simulink model "rc_coder"  (R2019b)
settings: Solver=FixedStepDiscrete  StartTime=0.0  StopTime=Inf  FixedStep=0.025  RelTol=1e-3  EnableMultiTasking=on
PreLoadFcn:
  | mdlname = bdroot;
  | oldFolder = cd(fileparts(which(mdlname)));
  | % cd ..\
  | 
  | load('./bus_type/bus_type.mat');
model workspace (MAT data in the model file):
  ADCDRES = Simulink.Parameter
  ADCDRES.Value = 65536
  ADCDRES.DataType = 'auto'
  ADCDRES.Dimensions = [1 1]
  ADCSRES = Simulink.Parameter
  ADCSRES.Value = 4096
  ADCSRES.DataType = 'auto'
  ADCSRES.Dimensions = [1 1]
  CLK = Simulink.Parameter
  CLK.Value = 200000000
  CLK.DataType = 'auto'
  CLK.Dimensions = [1 1]
  EncoderScaler = Simulink.Parameter
  EncoderScaler.Value = 1000
  EncoderScaler.DataType = 'auto'
  EncoderScaler.Dimensions = [1 1]
  GearBoxScaler = Simulink.Parameter
  GearBoxScaler.Value = 1
  GearBoxScaler.DataType = 'auto'
  GearBoxScaler.Dimensions = [1 1]
  Kd_T = Simulink.Parameter
  Kd_T.Value = 0.02
  Kd_T.DataType = 'auto'
  Kd_T.Dimensions = [1 1]
  Kd_theta = Simulink.Parameter
  Kd_theta.Value = 0
  Kd_theta.DataType = 'auto'
  Kd_theta.Dimensions = [1 1]
  Ki_T = Simulink.Parameter
  Ki_T.Value = 0
  Ki_T.DataType = 'auto'
  Ki_T.Dimensions = [1 1]
  Ki_theta = Simulink.Parameter
  Ki_theta.Value = 0.1
  Ki_theta.DataType = 'auto'
  Ki_theta.Dimensions = [1 1]
  Kp_T = Simulink.Parameter
  Kp_T.Value = 0.1
  Kp_T.DataType = 'auto'
  Kp_T.Dimensions = [1 1]
  Kp_theta = Simulink.Parameter
  Kp_theta.Value = 4
  Kp_theta.DataType = 'auto'
  Kp_theta.Dimensions = [1 1]
  LowerTempLimitHigh = Simulink.Parameter
  LowerTempLimitHigh.Value = 30
  LowerTempLimitHigh.DataType = 'auto'
  LowerTempLimitHigh.Dimensions = [1 1]
  LowerTempLimitLow = Simulink.Parameter
  LowerTempLimitLow.Value = 15
  LowerTempLimitLow.DataType = 'auto'
  LowerTempLimitLow.Dimensions = [1 1]
  MinMeasurableSpd = Simulink.Parameter
  MinMeasurableSpd.Value = 2
  MinMeasurableSpd.DataType = 'auto'
  MinMeasurableSpd.Dimensions = [1 1]
  ModePWM = Simulink.Parameter
  ModePWM.Value = 56
  ModePWM.DataType = 'single'
  ModePWM.Dimensions = [1 1]
  ModePosition = Simulink.Parameter
  ModePosition.Value = 53
  ModePosition.DataType = 'single'
  ModePosition.Dimensions = [1 1]
  ModePrecool = Simulink.Parameter
  ModePrecool.Value = 60
  ModePrecool.DataType = 'single'
  ModePrecool.Dimensions = [1 1]
  ModeTemp = Simulink.Parameter
  ModeTemp.Value = 55
  ModeTemp.DataType = 'single'
  ModeTemp.Dimensions = [1 1]
  PWMFreq = Simulink.Parameter
  PWMFreq.Value = 20
  PWMFreq.DataType = 'auto'
  PWMFreq.Dimensions = [1 1]
  QuadratureEncScaler = Simulink.Parameter
  QuadratureEncScaler.Value = 4
  QuadratureEncScaler.DataType = 'auto'
  QuadratureEncScaler.Dimensions = [1 1]
  S1DelaySeconds = Simulink.Parameter
  S1DelaySeconds.Value = 1
  S1DelaySeconds.DataType = 'auto'
  S1DelaySeconds.Dimensions = [1 1]
  S2DelaySeconds = Simulink.Parameter
  S2DelaySeconds.Value = 2
  S2DelaySeconds.DataType = 'auto'
  S2DelaySeconds.Dimensions = [1 1]
  S3DelaySeconds = Simulink.Parameter
  S3DelaySeconds.Value = 3
  S3DelaySeconds.DataType = 'auto'
  S3DelaySeconds.Dimensions = [1 1]
  S4DelaySeconds = Simulink.Parameter
  S4DelaySeconds.Value = 4
  S4DelaySeconds.DataType = 'auto'
  S4DelaySeconds.Dimensions = [1 1]
  SamplingR = Simulink.Parameter
  SamplingR.Value = 0.1
  SamplingR.DataType = 'auto'
  SamplingR.Dimensions = [1 1]
  StepSize = Simulink.Parameter
  StepSize.Value = 0.025
  StepSize.DataType = 'auto'
  StepSize.Dimensions = [1 1]
  TErrBand = Simulink.Parameter
  TErrBand.Value = 0.2
  TErrBand.DataType = 'auto'
  TErrBand.Dimensions = [1 1]
  ThetaErrBand = Simulink.Parameter
  ThetaErrBand.Value = 0.2
  ThetaErrBand.DataType = 'auto'
  ThetaErrBand.Dimensions = [1 1]
  VADCREF = Simulink.Parameter
  VADCREF.Value = 3
  VADCREF.DataType = 'auto'
  VADCREF.Dimensions = [1 1]
undefined symbols (not defined in the file or in its folder): DiscIntNeverNeededParam, Down, GPTRIP1SEL, GPTRIP2SEL, TZ1, TZ2, Up
libraries: simulink x21, c2802xlib x12, c2837xDlib x10, c280xlib x9, dspstat3 x8, dspfdesign x7, commutil2 x3, c2000lib x2
(part 1 of 4)
CloseFcn:
  | cd(oldFolder);
Description:
  | -> System Description <-
  | - Development environment:
  |     Matlab (version 2019b) with licence to
  |     - Simulink
  |     - Embedded Coder Support Package for Texas Instruments C2000 Processors
  |     - StateFlow
  | - Control board:
  |     TI LAUNCHXL F28379D
settings Model: SimulationMode=external  ExtModeTrigDuration=8  OrderedModelArguments=off  Creator=Quinn Ding  LastModifiedBy=Quinn
settings OptimizationCC: DefaultUnderspecifiedDataType=single  EnhancedBackFolding=on  PassReuseOutputArgsAs=Individual arguments  ZeroExternalMemoryAtStartup=off  MaxStackSize=1024  OptimizeBlockOrder=speed  DifferentSizesBufferReuse=on  OptimizationCustomize=off  DenormalBehavior=FlushToZero  EfficientTunableParamExpr=on
settings DebuggingCC: ParameterTunabilityLossMsg=error
settings HardwareCC: ProdBitPerChar=16  ProdBitPerInt=16  ProdBitPerPointer=32  ProdBitPerSizeT=32  ProdBitPerPtrDiffT=32  ProdLargestAtomicInteger=Integer  ProdLargestAtomicFloat=None  ProdWordSize=16  ProdLongLongMode=on  ProdHWDeviceType=Texas Instruments->C2000
settings SFSimCC: MATLABDynamicMemAlloc=off
settings RTWCC: SystemTargetFile=ert.tlc  HardwareBoard=TI Delfino F28379D LaunchPad  TLCOptions=-aInlineSetEventsForThisBaseRateFcn=TLC_FALSE -aSuppressMultiTaskScheduler=TLC_FALSE -aRateBasedStepFcn=1  TemplateMakefile=ert_default_tmf  Toolchain=Texas Instruments Code Composer Studio (C2000)  BuildConfiguration=Faster Runs  IncludeHyperlinkInReport=on
settings CodeAppCC: ForceParamTrailComments=on  IgnoreCustomStorageClasses=off  OperatorAnnotations=on  SimulinkDataObjDesc=on  SFDataObjDesc=on  InsertBlockDesc=on
settings ERTTargetCC: TargetLangStandard=C99 (ISO)  CodeReplacementLibrary=TI C28x  ExtModeStaticAllocSize=10000  RootIOFormat=Structure reference

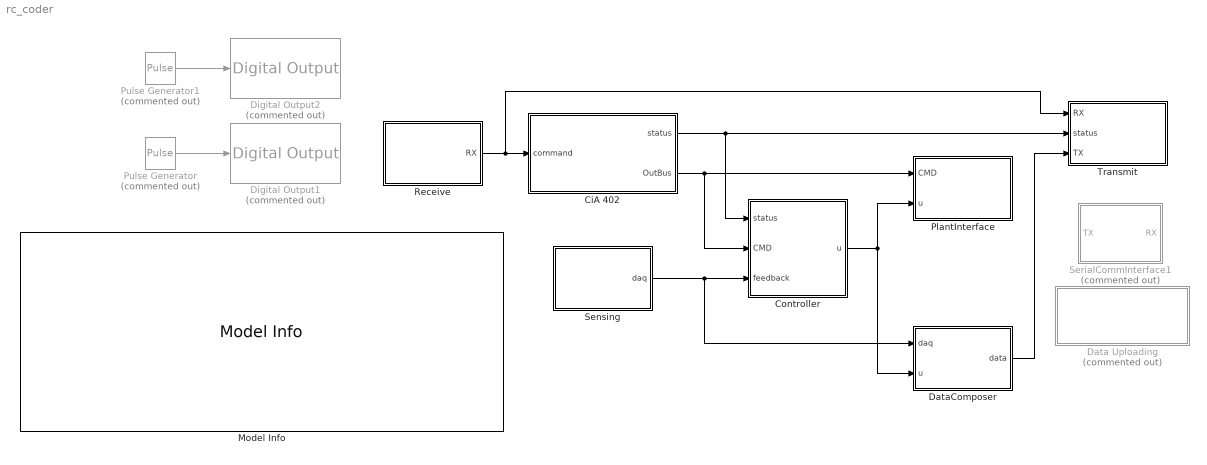
== system rc_coder ==
  CiA 402 : Stateflow chart  BlockKeywords=__PRM__SERIALIZED__DATA__:Stateflow Chart,Stateflow Diagram  TreatAsAtomicUnit=on
  Controller : Subsystem
  Data Uploading : Subsystem  Commented=on
      mask Display: disp('Data Uploading');
  DataComposer : Subsystem
  Digital Output1 : c2837xDlib/Digital Output  Commented=on  GPIO_Number=GPIO24~GPIO31  GPIO_Bit0=off  GPIO_BIT0_Toggle=off  GPIO_Bit1=off  GPIO_BIT1_Toggle=off  GPIO_Bit2=off  GPIO_BIT2_Toggle=off  GPIO_Bit3=off  GPIO_BIT3_Toggle=off  GPIO_Bit4=off  GPIO_BIT4_Toggle=off  GPIO_Bit5=off  GPIO_BIT5_Toggle=off  GPIO_Bit6=off  GPIO_BIT6_Toggle=off  GPIO_Bit7=on  GPIO_BIT7_Toggle=off
      settings: SourceProductName=Embedded Coder Support Package for Texas Instruments C2000 Processors  SourceProductBaseCode=TIC2000
  Digital Output2 : c2837xDlib/Digital Output  Commented=on  GPIO_Number=GPIO64~GPIO71  GPIO_Bit0=off  GPIO_BIT0_Toggle=off  GPIO_Bit1=off  GPIO_BIT1_Toggle=off  GPIO_Bit2=on  GPIO_BIT2_Toggle=off  GPIO_Bit3=off  GPIO_BIT3_Toggle=off  GPIO_Bit4=off  GPIO_BIT4_Toggle=off  GPIO_Bit5=off  GPIO_BIT5_Toggle=off  GPIO_Bit6=off  GPIO_BIT6_Toggle=off  GPIO_Bit7=off  GPIO_BIT7_Toggle=off
      settings: SourceProductName=Embedded Coder Support Package for Texas Instruments C2000 Processors  SourceProductBaseCode=TIC2000
  Model Info : simulink/Model-Wide Utilities/Model Info  Frame=on  DisplayStringWithTags=|  HorizontalTextAlignment=Left  LeftAlignmentValue=0.02
      | DSP controller coder %<ModelVersion> of SMA actuator.
      | 
      | Developed by %<Creator> at the Surgical Robotics & Instrumentation Laboratory, CUHK.
      | 
      | Last updated at %<LastModificationDate>.
      | 
      | %<Description>
  PlantInterface : Subsystem
  Pulse Generator : DiscretePulseGenerator  Commented=on  Period=10  PulseWidth=5  SampleTime=-1
  Pulse Generator1 : DiscretePulseGenerator  Commented=on  Period=10  PulseWidth=5  SampleTime=-1
  Receive : Subsystem
  Sensing : Subsystem
      mask Display: disp('Sensing');
  SerialCommInterface1 : Subsystem  Commented=on
  Transmit : Subsystem
  wires:
  DataComposer/1(data) -> Transmit/3(TX)
  Sensing/1(daq) -> DataComposer/1(daq), Controller/3(feedback)
  Pulse Generator/1 -> Digital Output1/1
  Controller/1(u) -> DataComposer/2(u), PlantInterface/2(u)
  CiA 402/2(OutBus) -> Controller/2(CMD), PlantInterface/1(CMD)
  Receive/1(RX) -> Transmit/1(RX), CiA 402/1(command)
  CiA 402/1(status) -> Transmit/2(status), Controller/1(status)
  Pulse Generator1/1 -> Digital Output2/1

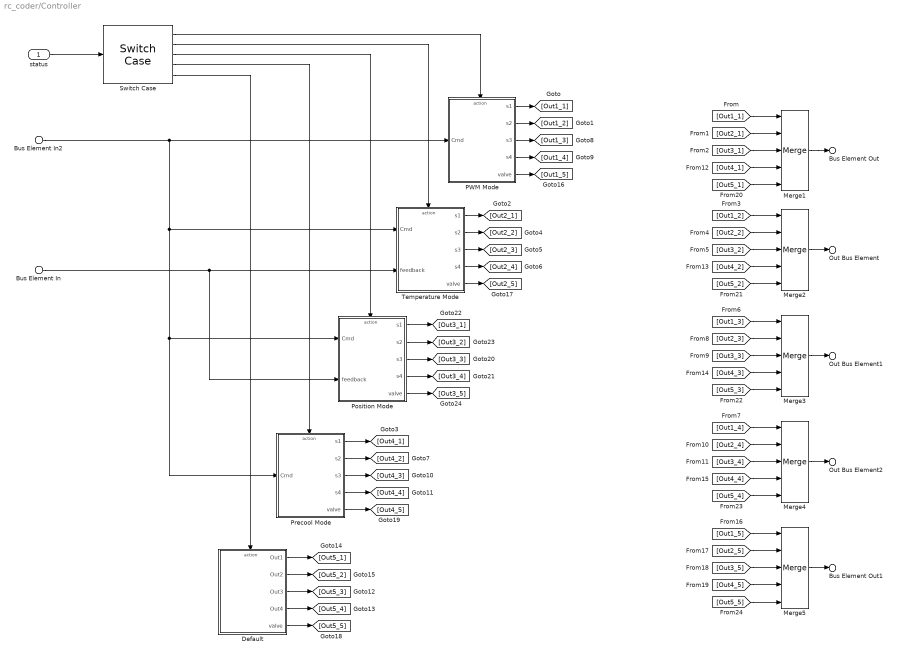
== system rc_coder/Controller ==
  status : Inport
  Bus Element In2 : Inport  Port=2  PortName=CMD
  Bus Element In : Inport  Port=3  PortName=feedback
  Default : Subsystem  TreatAsAtomicUnit=on
  Merge{1..5} (5 alike) : Merge  Inputs=5
  PWM Mode : Subsystem  TreatAsAtomicUnit=on
  Position Mode : Subsystem  TreatAsAtomicUnit=on
  Precool Mode : Subsystem  TreatAsAtomicUnit=on
  Switch Case : SwitchCase  CaseConditions={int32(ModePWM), int32(ModeTemp), int32(ModePosition), int32(ModePrecool)}
  Temperature Mode : Subsystem  TreatAsAtomicUnit=on
  Bus Element Out : Outport  PortName=u  Element=S1
  Out Bus Element : Outport  PortName=u  Element=S2
  Out Bus Element1 : Outport  PortName=u  Element=S3
  Out Bus Element2 : Outport  PortName=u  Element=S4
  Bus Element Out1 : Outport  PortName=u  Element=valveCmd
  wires:
  status/1 -> Switch Case/1
  Bus Element In2/1 -> PWM Mode/1(Cmd), Precool Mode/1(Cmd), Position Mode/1(Cmd), Temperature Mode/1(Cmd)
  [Out1_1] -> Merge1/1
  Switch Case/1 -> PWM Mode/Action
  Switch Case/2 -> Temperature Mode/Action
  Merge1/1 -> Bus Element Out/1
  [Out2_1] -> Merge1/2
  Merge2/1 -> Out Bus Element/1
  [Out2_2] -> Merge2/2
  Bus Element In/1 -> Position Mode/2(feedback), Temperature Mode/2(feedback)
  Merge3/1 -> Out Bus Element1/1
  Merge4/1 -> Out Bus Element2/1
  [Out1_3] -> Merge3/1
  [Out1_4] -> Merge4/1
  [Out2_3] -> Merge3/2
  [Out2_4] -> Merge4/2
  Switch Case/5 -> Default/Action
  [Out3_2] -> Merge2/3
  [Out3_3] -> Merge3/3
  [Out3_4] -> Merge4/3
  PWM Mode/1(s1) -> [Out1_1]
  PWM Mode/2(s2) -> [Out1_2]
  Temperature Mode/1(s1) -> [Out2_1]
  [Out3_1] -> Merge1/3
  Temperature Mode/2(s2) -> [Out2_2]
  Temperature Mode/3(s3) -> [Out2_3]
  Temperature Mode/4(s4) -> [Out2_4]
  [Out1_2] -> Merge2/1
  PWM Mode/3(s3) -> [Out1_3]
  PWM Mode/4(s4) -> [Out1_4]
  Switch Case/4 -> Precool Mode/Action
  [Out4_1] -> Merge1/4
  [Out4_2] -> Merge2/4
  [Out4_3] -> Merge3/4
  [Out4_4] -> Merge4/4
  Merge5/1 -> Bus Element Out1/1
  PWM Mode/5(valve) -> [Out1_5]
  [Out1_5] -> Merge5/1
  Temperature Mode/5(valve) -> [Out2_5]
  [Out2_5] -> Merge5/2
  [Out3_5] -> Merge5/3
  [Out4_5] -> Merge5/4
  Switch Case/3 -> Position Mode/Action
  Position Mode/2(s2) -> [Out3_2]
  Position Mode/1(s1) -> [Out3_1]
  Position Mode/3(s3) -> [Out3_3]
  Position Mode/5(valve) -> [Out3_5]
  Position Mode/4(s4) -> [Out3_4]
  Default/2(Out2) -> [Out5_2]
  Default/1(Out1) -> [Out5_1]
  Default/3(Out3) -> [Out5_3]
  Default/5(valve) -> [Out5_5]
  Default/4(Out4) -> [Out5_4]
  Precool Mode/3(s3) -> [Out4_3]
  Precool Mode/4(s4) -> [Out4_4]
  Precool Mode/2(s2) -> [Out4_2]
  Precool Mode/1(s1) -> [Out4_1]
  Precool Mode/5(valve) -> [Out4_5]
  [Out5_1] -> Merge1/5
  [Out5_2] -> Merge2/5
  [Out5_3] -> Merge3/5
  [Out5_4] -> Merge4/5
  [Out5_5] -> Merge5/5

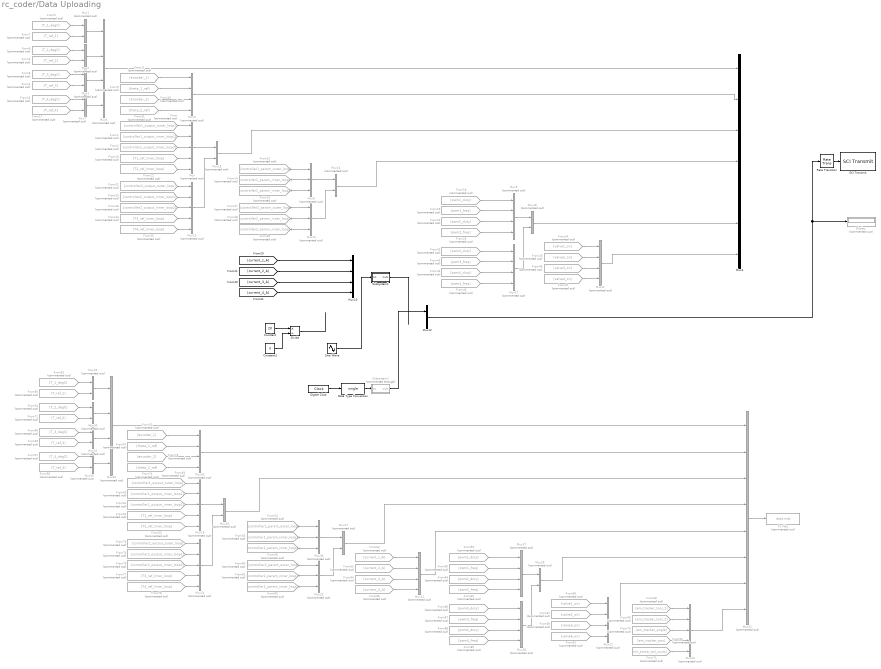
== system rc_coder/Data Uploading ==
  Constant : Constant  Value=20
  Constant1 : Constant  Value=3
  Data Type Conversion : DataTypeConversion  OutDataTypeStr=single
  Digital Clock : DigitalClock  SampleTime=0.001
  Display : Display  Commented=on
  Divide : Product  Inputs=*/
  From : From  Commented=on  GotoTag=controller1_output_outer_loop
  From1 : From  Commented=on  GotoTag=controller1_output_inner_loop1
  From10 : From  Commented=on  GotoTag=T1_ref_inner_loop
  From11 : From  Commented=on  GotoTag=encoder_1  TagVisibility=global
  From12 : From  Commented=on  GotoTag=T2_ref_inner_loop
  From13 : From  Commented=on  GotoTag=controller1_param_outer_loop
  From14 : From  Commented=on  GotoTag=controller1_param_inner_loop1
  From15 : From  Commented=on  GotoTag=controller1_param_inner_loop2
  From16 : From  Commented=on  GotoTag=T_4_degC
  From17 : From  Commented=on  GotoTag=T_ref_4
  From18 : From  Commented=on  GotoTag=pwm1_duty
  From19 : From  Commented=on  GotoTag=pwm1_freq
  From2 : From  Commented=on  GotoTag=controller1_output_inner_loop2
  From22 : From  Commented=on  GotoTag=pwm2_duty
  From23 : From  Commented=on  GotoTag=pwm2_freq
  From24 : From  Commented=on  GotoTag=valve1_on
  From25 : From  Commented=on  GotoTag=valve2_on
  From3 : From  Commented=on  GotoTag=T_ref_2
  From30 : From  Commented=on  GotoTag=encoder_2  TagVisibility=global
  From31 : From  Commented=on  GotoTag=theta_2_ref
  From32 : From  Commented=on  GotoTag=controller2_output_outer_loop
  From33 : From  Commented=on  GotoTag=controller2_output_inner_loop1
  From34 : From  Commented=on  GotoTag=T3_ref_inner_loop
  From35 : From  Commented=on  GotoTag=T4_ref_inner_loop
  From36 : From  Commented=on  GotoTag=controller2_output_inner_loop2
  From37 : From  Commented=on  GotoTag=controller2_param_outer_loop
  From38 : From  Commented=on  GotoTag=controller2_param_inner_loop1
  From39 : From  Commented=on  GotoTag=controller2_param_inner_loop2
  From4 : From  Commented=on  GotoTag=T_ref_3
  From42 : From  Commented=on  GotoTag=pwm3_duty
  From43 : From  Commented=on  GotoTag=pwm3_freq
  From44 : From  Commented=on  GotoTag=pwm4_duty
  From45 : From  Commented=on  GotoTag=pwm4_freq
  From46 : From  Commented=on  GotoTag=valve3_on
  From47 : From  Commented=on  GotoTag=valve4_on
  From49 : From  Commented=on  GotoTag=controller1_output_outer_loop  TagVisibility=global
  From5 : From  Commented=on  GotoTag=T_1_degC  TagVisibility=global
  From50 : From  Commented=on  GotoTag=controller1_output_inner_loop1  TagVisibility=global
  From51 : From  Commented=on  GotoTag=T1_ref_inner_loop  TagVisibility=global
  From52 : From  Commented=on  GotoTag=encoder_1  TagVisibility=global
  From53 : From  Commented=on  GotoTag=T2_ref_inner_loop  TagVisibility=global
  From54 : From  Commented=on  GotoTag=controller1_param_outer_loop  TagVisibility=global
  From55 : From  Commented=on  GotoTag=controller1_param_inner_loop1  TagVisibility=global
  From56 : From  Commented=on  GotoTag=controller1_param_inner_loop2  TagVisibility=global
  From57 : From  Commented=on  GotoTag=T_4_degC  TagVisibility=global
  From58 : From  Commented=on  GotoTag=T_ref_4  TagVisibility=global
  From59 : From  Commented=on  GotoTag=pwm1_duty  TagVisibility=global
  From6 : From  Commented=on  GotoTag=T_2_degC
  From60 : From  Commented=on  GotoTag=pwm1_freq  TagVisibility=global
  From61 : From  Commented=on  GotoTag=controller1_output_inner_loop2  TagVisibility=global
  From62 : From  Commented=on  GotoTag=current_1_A  TagVisibility=global
  From63 : From  Commented=on  GotoTag=current_2_A  TagVisibility=global
  From64 : From  Commented=on  GotoTag=pwm2_duty  TagVisibility=global
  From65 : From  Commented=on  GotoTag=pwm2_freq  TagVisibility=global
  From66 : From  Commented=on  GotoTag=valve1_on  TagVisibility=global
  From67 : From  Commented=on  GotoTag=valve2_on  TagVisibility=global
  From68 : From  Commented=on  GotoTag=em_tracker_tool_1  TagVisibility=global
  From69 : From  Commented=on  GotoTag=em_tracker_tool_2  TagVisibility=global
  From7 : From  Commented=on  GotoTag=T_ref_1
  From70 : From  Commented=on  GotoTag=em_tracker_angle  TagVisibility=global
  From71 : From  Commented=on  GotoTag=em_tracker_tool_counts  TagVisibility=global
  From72 : From  Commented=on  GotoTag=T_ref_2  TagVisibility=global
  From73 : From  Commented=on  GotoTag=encoder_2  TagVisibility=global
  From74 : From  Commented=on  GotoTag=theta_2_ref  TagVisibility=global
  From75 : From  Commented=on  GotoTag=controller2_output_outer_loop  TagVisibility=global
  From76 : From  Commented=on  GotoTag=controller2_output_inner_loop1  TagVisibility=global
  From77 : From  Commented=on  GotoTag=T3_ref_inner_loop  TagVisibility=global
  From78 : From  Commented=on  GotoTag=T4_ref_inner_loop  TagVisibility=global
  From79 : From  Commented=on  GotoTag=controller2_output_inner_loop2  TagVisibility=global
  From8 : From  Commented=on  GotoTag=T_3_degC
  From80 : From  Commented=on  GotoTag=controller2_param_outer_loop  TagVisibility=global
  From81 : From  Commented=on  GotoTag=controller2_param_inner_loop1  TagVisibility=global
  From82 : From  Commented=on  GotoTag=controller2_param_inner_loop2  TagVisibility=global
  From83 : From  Commented=on  GotoTag=T_ref_3  TagVisibility=global
  From84 : From  Commented=on  GotoTag=current_3_A  TagVisibility=global
  From85 : From  Commented=on  GotoTag=current_4_A  TagVisibility=global
  From86 : From  Commented=on  GotoTag=pwm3_duty  TagVisibility=global
  From87 : From  Commented=on  GotoTag=pwm3_freq  TagVisibility=global
  From88 : From  Commented=on  GotoTag=pwm4_duty  TagVisibility=global
  From89 : From  Commented=on  GotoTag=pwm4_freq  TagVisibility=global
  From9 : From  Commented=on  GotoTag=theta_1_ref
  From90 : From  Commented=on  GotoTag=valve3_on  TagVisibility=global
  From91 : From  Commented=on  GotoTag=valve4_on  TagVisibility=global
  From92 : From  Commented=on  GotoTag=em_tracker_pos  TagVisibility=global
  From93 : From  Commented=on  GotoTag=T_1_degC  TagVisibility=global
  From94 : From  Commented=on  GotoTag=T_2_degC  TagVisibility=global
  From95 : From  Commented=on  GotoTag=T_ref_1  TagVisibility=global
  From96 : From  Commented=on  GotoTag=T_3_degC  TagVisibility=global
  From97 : From  Commented=on  GotoTag=theta_1_ref  TagVisibility=global
  Mux{,13,19,23..24} (5 alike) : Mux  Commented=on  Inputs=5
  Mux{1..3,7,15..16,18,20,26..27,29..31,35} (14 alike) : Mux  Commented=on  Inputs=2
  Mux10 : Mux
  Mux{5..6,9,11,17,21..22,28,33..34,37} (11 alike) : Mux  Commented=on
  Mux12 : Mux  Inputs=2
  Mux{8,14,25,36} (4 alike) : Mux  Commented=on  Inputs=3
  Mux32 : Mux  Commented=on  Inputs=8
  Mux4 : Mux  Inputs=7
  Rate Transition : RateTransition  OutPortSampleTime=0.005
  SCI Transmit : c280xlib/SCI Transmit  sciModule=A  dataHead='S'  dataTail='\r'  postInterrupt=off  numFifo=1
      settings: SourceProductName=Embedded Coder Support Package for Texas Instruments C2000 Processors
  Sine Wave : Sin  SineType=Sample based  Amplitude=10  Samples=100  SampleTime=0.1
  Subsystem1 : Subsystem  mask(Convert float number to integer with controlled precision){f=1e1}
      mask prompts: f "factor"
      mask help:
      | Output = round(input * factor)
      |
      | Example:
      | input = 3.1415926, factor = 1e2
      | -->
      | output = 314
      mask Display: disp('cvt');
  Subsystem2 : Subsystem  Commented=through  mask(Convert float number to integer with controlled precision){f=1e3}
      mask prompts: f "factor"
      mask help:
      | Output = round(input * factor)
      |
      | Example:
      | input = 3.1415926, factor = 1e2
      | -->
      | output = 314
      mask Display: disp('cvt');
  To File1 : ToFile  Commented=on  Filename=data.mat  MatrixName=data
  wires:
  From/1 -> Mux/1
  From1/1 -> Mux/2
  From2/1 -> Mux/3
  Mux/1 -> Mux15/1
  From8/1 -> Mux3/1
  From4/1 -> Mux3/2
  Mux3/1 -> Mux6/3
  From6/1 -> Mux2/1
  From3/1 -> Mux2/2
  Mux1/1 -> Mux6/1
  From7/1 -> Mux1/2
  Mux2/1 -> Mux6/2
  From5/1 -> Mux1/1
  From9/1 -> Mux5/2
  From11/1 -> Mux5/1
  Mux5/1 -> Mux4/2
  From10/1 -> Mux/4
  From12/1 -> Mux/5
  Mux6/1 -> Mux4/1
  From17/1 -> Mux7/2
  From16/1 -> Mux7/1
  Mux7/1 -> Mux6/4
  From13/1 -> Mux8/1
  From14/1 -> Mux8/2
  From15/1 -> Mux8/3
  Mux8/1 -> Mux16/1
  From18/1 -> Mux9/1
  From19/1 -> Mux9/2
  Mux9/1 -> Mux18/1
  [current_2_A] -> Mux10/2
  Divide/1 -> ?
  From22/1 -> Mux9/3
  From23/1 -> Mux9/4
  From25/1 -> Mux11/2
  From24/1 -> Mux11/1
  Mux11/1 -> Mux4/7
  From30/1 -> Mux5/3
  From31/1 -> Mux5/4
  Mux13/1 -> Mux15/2
  From35/1 -> Mux13/5
  From33/1 -> Mux13/2
  From34/1 -> Mux13/4
  From36/1 -> Mux13/3
  From32/1 -> Mux13/1
  From37/1 -> Mux14/1
  From38/1 -> Mux14/2
  From39/1 -> Mux14/3
  Mux14/1 -> Mux16/2
  Mux15/1 -> Mux4/3
  Mux16/1 -> Mux4/4
  [current_3_A] -> Mux10/3
  [current_4_A] -> Mux10/4
  From45/1 -> Mux17/4
  From43/1 -> Mux17/2
  From44/1 -> Mux17/3
  From42/1 -> Mux17/1
  Mux17/1 -> Mux18/2
  Mux18/1 -> Mux4/6
  From46/1 -> Mux11/3
  From47/1 -> Mux11/4
  From84/1 -> Mux21/3
  From59/1 -> Mux37/1
  From92/1 -> Mux23/4
  Mux29/1 -> Mux32/6
  From57/1 -> Mux35/1
  Mux32/1 -> To File1/1
  Mux37/1 -> Mux29/1
  From87/1 -> Mux28/2
  Mux25/1 -> Mux27/2
  From95/1 -> Mux20/2
  From90/1 -> Mux22/3
  From79/1 -> Mux24/3
  From81/1 -> Mux25/2
  From89/1 -> Mux28/4
  From53/1 -> Mux19/5
  From62/1 -> Mux21/1
  Mux28/1 -> Mux29/2
  Mux24/1 -> Mux26/2
  From85/1 -> Mux21/4
  From96/1 -> Mux31/1
  From75/1 -> Mux24/1
  From68/1 -> Mux23/1
  Mux22/1 -> Mux32/7
  From66/1 -> Mux22/1
  Mux33/1 -> Mux32/2
  From97/1 -> Mux33/2
  From91/1 -> Mux22/4
  From77/1 -> Mux24/4
  From73/1 -> Mux33/3
  From78/1 -> Mux24/5
  From69/1 -> Mux23/2
  Mux23/1 -> Mux32/8
  From67/1 -> Mux22/2
  From86/1 -> Mux28/1
  From52/1 -> Mux33/1
  Mux21/1 -> Mux32/5
  From65/1 -> Mux37/4
  From58/1 -> Mux35/2
  From54/1 -> Mux36/1
  From74/1 -> Mux33/4
  Mux30/1 -> Mux34/2
  Mux36/1 -> Mux27/1
  From55/1 -> Mux36/2
  From70/1 -> Mux23/3
  From71/1 -> Mux23/5
  From64/1 -> Mux37/3
  From56/1 -> Mux36/3
  From76/1 -> Mux24/2
  From63/1 -> Mux21/2
  From60/1 -> Mux37/2
  Mux34/1 -> Mux32/1
  Mux35/1 -> Mux34/4
  Mux19/1 -> Mux26/1
  From61/1 -> Mux19/3
  Mux27/1 -> Mux32/4
  Mux31/1 -> Mux34/3
  From80/1 -> Mux25/1
  From50/1 -> Mux19/2
  From94/1 -> Mux30/1
  From72/1 -> Mux30/2
  Mux26/1 -> Mux32/3
  From51/1 -> Mux19/4
  From82/1 -> Mux25/3
  From88/1 -> Mux28/3
  From83/1 -> Mux31/2
  From93/1 -> Mux20/1
  From49/1 -> Mux19/1
  Mux20/1 -> Mux34/1
  Mux12/1 -> Rate Transition/1, Display/1
  [current_1_A] -> Mux10/1
  Constant1/1 -> Divide/2
  Constant/1 -> Divide/1
  Subsystem1/1(Out1) -> ?
  Sine Wave/1 -> Subsystem1/1(In1)
  Rate Transition/1 -> SCI Transmit/1
  Digital Clock/1 -> Data Type Conversion/1
  Subsystem2/1(Out1) -> Mux12/1
  Data Type Conversion/1 -> Subsystem2/1(In1)

== system rc_coder/DataComposer ==
  daq1 : Inport  PortName=daq
  Bus Element In : Inport  Port=2  PortName=u  Element=valveCmd
  ElapsedTime : Subsystem
  Mux : Mux  Inputs=3
  SensorData7 : Subsystem
  data : Outport
  wires:
  daq1/1 -> SensorData7/1(daq)
  SensorData7/1(Out2) -> Mux/2
  Mux/1 -> data/1
  Bus Element In/1 -> Mux/3
  ElapsedTime/1(in format) -> Mux/1

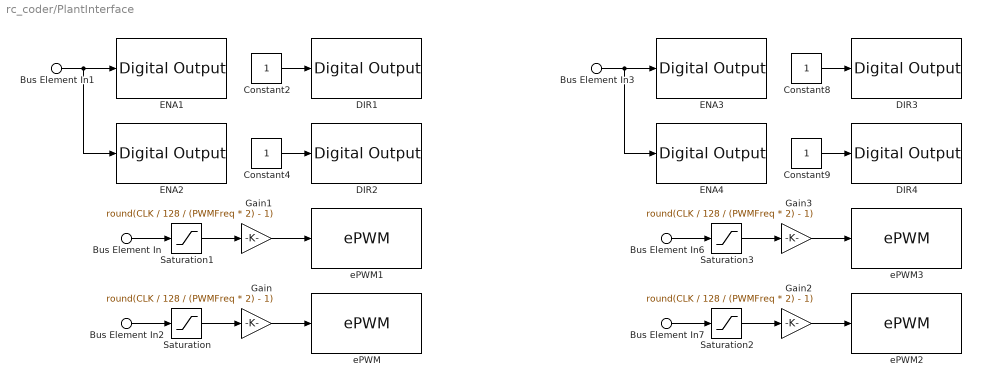
== system rc_coder/PlantInterface ==
  Bus Element In1 : Inport  PortName=CMD  Element=EnableActr1
  Bus Element In3 : Inport  PortName=CMD  Element=EnableActr2
  Bus Element In : Inport  Port=2  PortName=u  Element=S1
  Bus Element In2 : Inport  Port=2  PortName=u  Element=S2
  Bus Element In6 : Inport  Port=2  PortName=u  Element=S3
  Bus Element In7 : Inport  Port=2  PortName=u  Element=S4
  Constant{2,4,8..9} (4 alike) : Constant
  DIR1 : c2837xDlib/Digital Output  GPIO_Number=GPIO120~GPIO127  GPIO_Bit0=off  GPIO_BIT0_Toggle=off  GPIO_Bit1=off  GPIO_BIT1_Toggle=off  GPIO_Bit2=off  GPIO_BIT2_Toggle=off  GPIO_Bit3=on  GPIO_BIT3_Toggle=off  GPIO_Bit4=off  GPIO_BIT4_Toggle=off  GPIO_Bit5=off  GPIO_BIT5_Toggle=off  GPIO_Bit6=off  GPIO_BIT6_Toggle=off  GPIO_Bit7=off  GPIO_BIT7_Toggle=off
      settings: SourceProductName=Embedded Coder Support Package for Texas Instruments C2000 Processors  SourceProductBaseCode=TIC2000
  DIR2 : c2837xDlib/Digital Output  GPIO_Number=GPIO56~GPIO63  GPIO_Bit0=off  GPIO_BIT0_Toggle=off  GPIO_Bit1=off  GPIO_BIT1_Toggle=off  GPIO_Bit2=on  GPIO_BIT2_Toggle=off  GPIO_Bit3=off  GPIO_BIT3_Toggle=off  GPIO_Bit4=off  GPIO_BIT4_Toggle=off  GPIO_Bit5=off  GPIO_BIT5_Toggle=off  GPIO_Bit6=off  GPIO_BIT6_Toggle=off  GPIO_Bit7=off  GPIO_BIT7_Toggle=off
      settings: SourceProductName=Embedded Coder Support Package for Texas Instruments C2000 Processors  SourceProductBaseCode=TIC2000
  DIR3 : c2837xDlib/Digital Output  GPIO_Number=GPIO120~GPIO127  GPIO_Bit0=off  GPIO_BIT0_Toggle=off  GPIO_Bit1=off  GPIO_BIT1_Toggle=off  GPIO_Bit2=off  GPIO_BIT2_Toggle=off  GPIO_Bit3=off  GPIO_BIT3_Toggle=off  GPIO_Bit4=on  GPIO_BIT4_Toggle=off  GPIO_Bit5=off  GPIO_BIT5_Toggle=off  GPIO_Bit6=off  GPIO_BIT6_Toggle=off  GPIO_Bit7=off  GPIO_BIT7_Toggle=off
      settings: SourceProductName=Embedded Coder Support Package for Texas Instruments C2000 Processors  SourceProductBaseCode=TIC2000
  DIR4 : c2837xDlib/Digital Output  GPIO_Number=GPIO24~GPIO31  GPIO_Bit0=off  GPIO_BIT0_Toggle=off  GPIO_Bit1=off  GPIO_BIT1_Toggle=off  GPIO_Bit2=off  GPIO_BIT2_Toggle=off  GPIO_Bit3=off  GPIO_BIT3_Toggle=off  GPIO_Bit4=off  GPIO_BIT4_Toggle=off  GPIO_Bit5=on  GPIO_BIT5_Toggle=off  GPIO_Bit6=off  GPIO_BIT6_Toggle=off  GPIO_Bit7=off  GPIO_BIT7_Toggle=off
      settings: SourceProductName=Embedded Coder Support Package for Texas Instruments C2000 Processors  SourceProductBaseCode=TIC2000
  ENA1 : c2837xDlib/Digital Output  GPIO_Number=GPIO56~GPIO63  GPIO_Bit0=off  GPIO_BIT0_Toggle=off  GPIO_Bit1=off  GPIO_BIT1_Toggle=off  GPIO_Bit2=off  GPIO_BIT2_Toggle=off  GPIO_Bit3=off  GPIO_BIT3_Toggle=off  GPIO_Bit4=off  GPIO_BIT4_Toggle=off  GPIO_Bit5=on  GPIO_BIT5_Toggle=off  GPIO_Bit6=off  GPIO_BIT6_Toggle=off  GPIO_Bit7=off  GPIO_BIT7_Toggle=off
      settings: SourceProductName=Embedded Coder Support Package for Texas Instruments C2000 Processors  SourceProductBaseCode=TIC2000
  ENA2 : c2837xDlib/Digital Output  GPIO_Number=GPIO120~GPIO127  GPIO_Bit0=off  GPIO_BIT0_Toggle=off  GPIO_Bit1=off  GPIO_BIT1_Toggle=off  GPIO_Bit2=on  GPIO_BIT2_Toggle=off  GPIO_Bit3=off  GPIO_BIT3_Toggle=off  GPIO_Bit4=off  GPIO_BIT4_Toggle=off  GPIO_Bit5=off  GPIO_BIT5_Toggle=off  GPIO_Bit6=off  GPIO_BIT6_Toggle=off  GPIO_Bit7=off  GPIO_BIT7_Toggle=off
      settings: SourceProductName=Embedded Coder Support Package for Texas Instruments C2000 Processors  SourceProductBaseCode=TIC2000
  ENA3 : c2837xDlib/Digital Output  GPIO_Number=GPIO56~GPIO63  GPIO_Bit0=off  GPIO_BIT0_Toggle=off  GPIO_Bit1=off  GPIO_BIT1_Toggle=off  GPIO_Bit2=off  GPIO_BIT2_Toggle=off  GPIO_Bit3=on  GPIO_BIT3_Toggle=off  GPIO_Bit4=off  GPIO_BIT4_Toggle=off  GPIO_Bit5=off  GPIO_BIT5_Toggle=off  GPIO_Bit6=off  GPIO_BIT6_Toggle=off  GPIO_Bit7=off  GPIO_BIT7_Toggle=off
      settings: SourceProductName=Embedded Coder Support Package for Texas Instruments C2000 Processors  SourceProductBaseCode=TIC2000
  ENA4 : c2837xDlib/Digital Output  GPIO_Number=GPIO120~GPIO127  GPIO_Bit0=off  GPIO_BIT0_Toggle=off  GPIO_Bit1=off  GPIO_BIT1_Toggle=off  GPIO_Bit2=off  GPIO_BIT2_Toggle=off  GPIO_Bit3=off  GPIO_BIT3_Toggle=off  GPIO_Bit4=off  GPIO_BIT4_Toggle=off  GPIO_Bit5=on  GPIO_BIT5_Toggle=off  GPIO_Bit6=off  GPIO_BIT6_Toggle=off  GPIO_Bit7=off  GPIO_BIT7_Toggle=off
      settings: SourceProductName=Embedded Coder Support Package for Texas Instruments C2000 Processors  SourceProductBaseCode=TIC2000
  Gain{,1..3} (4 alike) : Gain  Gain=round(CLK / 128 / (PWMFreq * 2) - 1)
  Saturation{,1..3} (4 alike) : Saturate  UpperLimit=0.99  LowerLimit=0
  ePWM : c2802xlib/ePWM  useModule=ePWM1  ePWMxLINKTBPRD=Not Linked  periodUnits=Clock cycles  timerSource=Specify via dialog  timerPeriod_clk=round(CLK / 128 / (PWMFreq * 2) - 1)  timerPeriod_sec=0.0001  tbshadow=Counter equals to zero  countingMode=Up-Down  phaseActiveEnable=Disable  phaseDirection=Count down after sync  phaseActive=0  synchronizationEnable=off  dcaevt1Sync=off  dcbevt1Sync=off  synchronizationOption=Disable  clockPrescale=64  HSclockPrescale=1  enswap=off  ePWMxAStatus=on  ePWMxAactionLogic1=Set  ePWMxAactionLogic2=Clear  ePWMxAactionLogic3=Clear  ePWMxAactionLogic4=Set  ePWMxAactionLogic5=Do nothing  ePWMxAactionLogic6=Do nothing  ePWMxALoadMode=Load on counter equals to zero (CTR=Zero)  ePWMxACSFenable=off  ePWMxACSFvalue=Forcing disable  ePWMxASFreload=Zero  ePWMxBStatus=off  ePWMxBactionLogic1=Set  ePWMxBactionLogic2=Clear  ePWMxBactionLogic3=Do nothing  ePWMxBactionLogic4=Do nothing  ePWMxBactionLogic5=Clear  ePWMxBactionLogic6=Set  ePWMxBLoadMode=Load on counter equals to zero (CTR=Zero)  ePWMxBCSFenable=off  ePWMxBCSFvalue=Forcing disable  ePWMxBSFreload=Zero  ePWNxBOutWay=off  ePWMxLINKCMPA=Not Linked  CMPAUnits=Clock cycles  CMPASource=Input port  CMPAValue_per=50  CMPAValue_clk=32000  enCMPAshadow=Counter equals to zero  ePWMxLINKCMPB=Not Linked  CMPBUnits=Clock cycles  CMPBSource=Specify via dialog  CMPBValue_per=50  CMPBValue_clk=32000  enCMPBshadow=Counter equals to zero  ePWMxLINKCMPC=Not Linked  CMPCUnits=Clock cycles  CMPCSource=Specify via dialog  CMPCValue_per=50  CMPCValue_clk=32000  enCMPCshadow=Counter equals to zero  ePWMxLINKCMPD=Not Linked  CMPDUnits=Clock cycles  CMPDSource=Specify via dialog  CMPDValue_per=50  CMPDValue_clk=32000  enCMPDshadow=Counter equals to zero  enableDBePWMxA=off  enableDBePWMxB=off  enhalfcycle=off  DBpolarity=Active high (AH)  DBedgeDelay=Positive  DBSource_ePWMxA=ePWMxA  DBSource_ePWMxB=ePWMxA  DBperiodSource=Specify via dialog  REDperiod=0  FEDperiod=0  adcstartModuleA=off  adcrequestEventA=First event  adcstartEventA=Digital Compare Module A Event 1 start of conversion (DCAEVT1.soc)  adcstartEventA_type2=Digital Compare Module A Event 1 start of conversion (DCAEVT1.soc)  adcstartModuleB=off  adcrequestEventB=First event  adcstartEventB=Counter equals to zero (CTR=Zero)  adcstartEventB_type2=Counter equals to zero (CTR=Zero)  intEn=off  intPrd=First event  intSel=Counter equals to zero (CTR=Zero)  intSel_type2=Counter equals to zero (CTR=Zero)  hrpe=off  enHRPWM=off  HRPWM_LoadMode=Counter equals to period (CTR=PRD)  HRPWM_CTLMode=Duty or Period control mode  HRPWM_EDGMode=Both edge  hrpeb=off  enHRPWMB=off  HRPWM_LoadModeB=Counter equals to zero (CTR=ZERO)  HRPWM_CTLModeB=Duty or Period control mode  HRPWM_EDGModeB=Both edge  enSFO=on  enautoconv=on  chopperEnable=off  chopperFrequency=1  chopperFirstwidth=1  chopperDuty=12.5%  tripZonesource=Specify via dialog  tzselOSHT1=off  tzselOSHT2=off  tzselOSHT3=off  tzselOSHDCAEV1=off  tzselOSHDCBEV1=off  tzselCBC1=off  tzselCBC2=off  tzselCBC3=off  tzselCBCDCAEV2=off  tzselCBCDCBEV2=off  tzselOSHT4=off  tzselOSHT5=off  tzselOSHT6=off  tzselCBC4=off  tzselCBC5=off  tzselCBC6=off  enTzOstIntr=off  enTzCbcIntr=off  enTzDCAEVT1Intr=off  enTzDCAEVT2Intr=off  enTzDCBEVT1Intr=off  enTzDCBEVT2Intr=off  ePWMxAforced=No action  ePWMxBforced=No action  DCAEVT1forced=No action  DCBEVT1forced=No action  DCAEVT2forced=No action  DCBEVT2forced=No action  dcah=Trip Zone 1 input (TZ1)  dcal=Trip Zone 2 input (TZ2)  dcbh=Trip Zone 1 input (TZ1)  dcbl=Trip Zone 2 input (TZ2)  dcah_type2=GPTRIP1SEL/(TZ1)  dcal_type2=GPTRIP2SEL/(TZ2)  dcbh_type2=GPTRIP1SEL/(TZ1)  dcbl_type2=GPTRIP2SEL/(TZ2)  gendcaevt1=Event disabled  gendcaevt2=Event disabled  gendcbevt1=Event disabled  gendcbevt2=Event disabled  dcaevt1src=DCAEVT1 with sync  dcaevt2src=DCAEVT2 with sync  dcbevt1src=DCBEVT1 with sync  dcbevt2src=DCBEVT2 with sync  pulsesel=Counter equals to zero (CTR=Zero)  blankinv=off  blankoffset=0  blankwidth=0  evsrcsel=Filtered version of DCAEVT1 (DCAEVT1FILT)  encape=off  PwmType=C2000_Type4
      settings: SourceProductName=Embedded Coder Support Package for Texas Instruments C2000 Processors
  ePWM1 : c2802xlib/ePWM  useModule=ePWM2  ePWMxLINKTBPRD=Not Linked  periodUnits=Clock cycles  timerSource=Specify via dialog  timerPeriod_clk=round(CLK / 128 / (PWMFreq * 2) - 1)  timerPeriod_sec=0.0001  tbshadow=Counter equals to zero  countingMode=Up-Down  phaseActiveEnable=Disable  phaseDirection=Count down after sync  phaseActive=0  synchronizationEnable=off  dcaevt1Sync=off  dcbevt1Sync=off  synchronizationOption=Disable  clockPrescale=64  HSclockPrescale=1  enswap=off  ePWMxAStatus=on  ePWMxAactionLogic1=Set  ePWMxAactionLogic2=Clear  ePWMxAactionLogic3=Clear  ePWMxAactionLogic4=Set  ePWMxAactionLogic5=Do nothing  ePWMxAactionLogic6=Do nothing  ePWMxALoadMode=Load on counter equals to zero (CTR=Zero)  ePWMxACSFenable=off  ePWMxACSFvalue=Forcing disable  ePWMxASFreload=Zero  ePWMxBStatus=off  ePWMxBactionLogic1=Set  ePWMxBactionLogic2=Clear  ePWMxBactionLogic3=Do nothing  ePWMxBactionLogic4=Do nothing  ePWMxBactionLogic5=Clear  ePWMxBactionLogic6=Set  ePWMxBLoadMode=Load on counter equals to zero (CTR=Zero)  ePWMxBCSFenable=off  ePWMxBCSFvalue=Forcing disable  ePWMxBSFreload=Zero  ePWNxBOutWay=off  ePWMxLINKCMPA=Not Linked  CMPAUnits=Clock cycles  CMPASource=Input port  CMPAValue_per=50  CMPAValue_clk=32000  enCMPAshadow=Counter equals to zero  ePWMxLINKCMPB=Not Linked  CMPBUnits=Clock cycles  CMPBSource=Specify via dialog  CMPBValue_per=50  CMPBValue_clk=32000  enCMPBshadow=Counter equals to zero  ePWMxLINKCMPC=Not Linked  CMPCUnits=Clock cycles  CMPCSource=Specify via dialog  CMPCValue_per=50  CMPCValue_clk=32000  enCMPCshadow=Counter equals to zero  ePWMxLINKCMPD=Not Linked  CMPDUnits=Clock cycles  CMPDSource=Specify via dialog  CMPDValue_per=50  CMPDValue_clk=32000  enCMPDshadow=Counter equals to zero  enableDBePWMxA=off  enableDBePWMxB=off  enhalfcycle=off  DBpolarity=Active high (AH)  DBedgeDelay=Positive  DBSource_ePWMxA=ePWMxA  DBSource_ePWMxB=ePWMxA  DBperiodSource=Specify via dialog  REDperiod=0  FEDperiod=0  adcstartModuleA=off  adcrequestEventA=First event  adcstartEventA=Digital Compare Module A Event 1 start of conversion (DCAEVT1.soc)  adcstartEventA_type2=Digital Compare Module A Event 1 start of conversion (DCAEVT1.soc)  adcstartModuleB=off  adcrequestEventB=First event  adcstartEventB=Counter equals to zero (CTR=Zero)  adcstartEventB_type2=Counter equals to zero (CTR=Zero)  intEn=off  intPrd=First event  intSel=Counter equals to zero (CTR=Zero)  intSel_type2=Counter equals to zero (CTR=Zero)  hrpe=off  enHRPWM=off  HRPWM_LoadMode=Counter equals to period (CTR=PRD)  HRPWM_CTLMode=Duty or Period control mode  HRPWM_EDGMode=Both edge  hrpeb=off  enHRPWMB=off  HRPWM_LoadModeB=Counter equals to zero (CTR=ZERO)  HRPWM_CTLModeB=Duty or Period control mode  HRPWM_EDGModeB=Both edge  enSFO=on  enautoconv=on  chopperEnable=off  chopperFrequency=1  chopperFirstwidth=1  chopperDuty=12.5%  tripZonesource=Specify via dialog  tzselOSHT1=off  tzselOSHT2=off  tzselOSHT3=off  tzselOSHDCAEV1=off  tzselOSHDCBEV1=off  tzselCBC1=off  tzselCBC2=off  tzselCBC3=off  tzselCBCDCAEV2=off  tzselCBCDCBEV2=off  tzselOSHT4=off  tzselOSHT5=off  tzselOSHT6=off  tzselCBC4=off  tzselCBC5=off  tzselCBC6=off  enTzOstIntr=off  enTzCbcIntr=off  enTzDCAEVT1Intr=off  enTzDCAEVT2Intr=off  enTzDCBEVT1Intr=off  enTzDCBEVT2Intr=off  ePWMxAforced=No action  ePWMxBforced=No action  DCAEVT1forced=No action  DCBEVT1forced=No action  DCAEVT2forced=No action  DCBEVT2forced=No action  dcah=Trip Zone 1 input (TZ1)  dcal=Trip Zone 2 input (TZ2)  dcbh=Trip Zone 1 input (TZ1)  dcbl=Trip Zone 2 input (TZ2)  dcah_type2=GPTRIP1SEL/(TZ1)  dcal_type2=GPTRIP2SEL/(TZ2)  dcbh_type2=GPTRIP1SEL/(TZ1)  dcbl_type2=GPTRIP2SEL/(TZ2)  gendcaevt1=Event disabled  gendcaevt2=Event disabled  gendcbevt1=Event disabled  gendcbevt2=Event disabled  dcaevt1src=DCAEVT1 with sync  dcaevt2src=DCAEVT2 with sync  dcbevt1src=DCBEVT1 with sync  dcbevt2src=DCBEVT2 with sync  pulsesel=Counter equals to zero (CTR=Zero)  blankinv=off  blankoffset=0  blankwidth=0  evsrcsel=Filtered version of DCAEVT1 (DCAEVT1FILT)  encape=off  PwmType=C2000_Type4
      settings: SourceProductName=Embedded Coder Support Package for Texas Instruments C2000 Processors
  ePWM2 : c2802xlib/ePWM  useModule=ePWM3  ePWMxLINKTBPRD=Not Linked  periodUnits=Clock cycles  timerSource=Specify via dialog  timerPeriod_clk=round(CLK / 128 / (PWMFreq * 2) - 1)  timerPeriod_sec=0.0001  tbshadow=Counter equals to zero  countingMode=Up-Down  phaseActiveEnable=Disable  phaseDirection=Count down after sync  phaseActive=0  synchronizationEnable=off  dcaevt1Sync=off  dcbevt1Sync=off  synchronizationOption=Disable  clockPrescale=64  HSclockPrescale=1  enswap=off  ePWMxAStatus=on  ePWMxAactionLogic1=Set  ePWMxAactionLogic2=Clear  ePWMxAactionLogic3=Clear  ePWMxAactionLogic4=Set  ePWMxAactionLogic5=Do nothing  ePWMxAactionLogic6=Do nothing  ePWMxALoadMode=Load on counter equals to zero (CTR=Zero)  ePWMxACSFenable=off  ePWMxACSFvalue=Forcing disable  ePWMxASFreload=Zero  ePWMxBStatus=off  ePWMxBactionLogic1=Set  ePWMxBactionLogic2=Clear  ePWMxBactionLogic3=Do nothing  ePWMxBactionLogic4=Do nothing  ePWMxBactionLogic5=Clear  ePWMxBactionLogic6=Set  ePWMxBLoadMode=Load on counter equals to zero (CTR=Zero)  ePWMxBCSFenable=off  ePWMxBCSFvalue=Forcing disable  ePWMxBSFreload=Zero  ePWNxBOutWay=off  ePWMxLINKCMPA=Not Linked  CMPAUnits=Clock cycles  CMPASource=Input port  CMPAValue_per=50  CMPAValue_clk=32000  enCMPAshadow=Counter equals to zero  ePWMxLINKCMPB=Not Linked  CMPBUnits=Clock cycles  CMPBSource=Specify via dialog  CMPBValue_per=50  CMPBValue_clk=32000  enCMPBshadow=Counter equals to zero  ePWMxLINKCMPC=Not Linked  CMPCUnits=Clock cycles  CMPCSource=Specify via dialog  CMPCValue_per=50  CMPCValue_clk=32000  enCMPCshadow=Counter equals to zero  ePWMxLINKCMPD=Not Linked  CMPDUnits=Clock cycles  CMPDSource=Specify via dialog  CMPDValue_per=50  CMPDValue_clk=32000  enCMPDshadow=Counter equals to zero  enableDBePWMxA=off  enableDBePWMxB=off  enhalfcycle=off  DBpolarity=Active high (AH)  DBedgeDelay=Positive  DBSource_ePWMxA=ePWMxA  DBSource_ePWMxB=ePWMxA  DBperiodSource=Specify via dialog  REDperiod=0  FEDperiod=0  adcstartModuleA=off  adcrequestEventA=First event  adcstartEventA=Digital Compare Module A Event 1 start of conversion (DCAEVT1.soc)  adcstartEventA_type2=Digital Compare Module A Event 1 start of conversion (DCAEVT1.soc)  adcstartModuleB=off  adcrequestEventB=First event  adcstartEventB=Counter equals to zero (CTR=Zero)  adcstartEventB_type2=Counter equals to zero (CTR=Zero)  intEn=off  intPrd=First event  intSel=Counter equals to zero (CTR=Zero)  intSel_type2=Counter equals to zero (CTR=Zero)  hrpe=off  enHRPWM=off  HRPWM_LoadMode=Counter equals to period (CTR=PRD)  HRPWM_CTLMode=Duty or Period control mode  HRPWM_EDGMode=Both edge  hrpeb=off  enHRPWMB=off  HRPWM_LoadModeB=Counter equals to zero (CTR=ZERO)  HRPWM_CTLModeB=Duty or Period control mode  HRPWM_EDGModeB=Both edge  enSFO=on  enautoconv=on  chopperEnable=off  chopperFrequency=1  chopperFirstwidth=1  chopperDuty=12.5%  tripZonesource=Specify via dialog  tzselOSHT1=off  tzselOSHT2=off  tzselOSHT3=off  tzselOSHDCAEV1=off  tzselOSHDCBEV1=off  tzselCBC1=off  tzselCBC2=off  tzselCBC3=off  tzselCBCDCAEV2=off  tzselCBCDCBEV2=off  tzselOSHT4=off  tzselOSHT5=off  tzselOSHT6=off  tzselCBC4=off  tzselCBC5=off  tzselCBC6=off  enTzOstIntr=off  enTzCbcIntr=off  enTzDCAEVT1Intr=off  enTzDCAEVT2Intr=off  enTzDCBEVT1Intr=off  enTzDCBEVT2Intr=off  ePWMxAforced=No action  ePWMxBforced=No action  DCAEVT1forced=No action  DCBEVT1forced=No action  DCAEVT2forced=No action  DCBEVT2forced=No action  dcah=Trip Zone 1 input (TZ1)  dcal=Trip Zone 2 input (TZ2)  dcbh=Trip Zone 1 input (TZ1)  dcbl=Trip Zone 2 input (TZ2)  dcah_type2=GPTRIP1SEL/(TZ1)  dcal_type2=GPTRIP2SEL/(TZ2)  dcbh_type2=GPTRIP1SEL/(TZ1)  dcbl_type2=GPTRIP2SEL/(TZ2)  gendcaevt1=Event disabled  gendcaevt2=Event disabled  gendcbevt1=Event disabled  gendcbevt2=Event disabled  dcaevt1src=DCAEVT1 with sync  dcaevt2src=DCAEVT2 with sync  dcbevt1src=DCBEVT1 with sync  dcbevt2src=DCBEVT2 with sync  pulsesel=Counter equals to zero (CTR=Zero)  blankinv=off  blankoffset=0  blankwidth=0  evsrcsel=Filtered version of DCAEVT1 (DCAEVT1FILT)  encape=off  PwmType=C2000_Type4
      settings: SourceProductName=Embedded Coder Support Package for Texas Instruments C2000 Processors
  ePWM3 : c2802xlib/ePWM  useModule=ePWM4  ePWMxLINKTBPRD=Not Linked  periodUnits=Clock cycles  timerSource=Specify via dialog  timerPeriod_clk=round(CLK / 128 / (PWMFreq * 2) - 1)  timerPeriod_sec=0.0001  tbshadow=Counter equals to zero  countingMode=Up-Down  phaseActiveEnable=Disable  phaseDirection=Count down after sync  phaseActive=0  synchronizationEnable=off  dcaevt1Sync=off  dcbevt1Sync=off  synchronizationOption=Disable  clockPrescale=64  HSclockPrescale=1  enswap=off  ePWMxAStatus=on  ePWMxAactionLogic1=Set  ePWMxAactionLogic2=Clear  ePWMxAactionLogic3=Clear  ePWMxAactionLogic4=Set  ePWMxAactionLogic5=Do nothing  ePWMxAactionLogic6=Do nothing  ePWMxALoadMode=Load on counter equals to zero (CTR=Zero)  ePWMxACSFenable=off  ePWMxACSFvalue=Forcing disable  ePWMxASFreload=Zero  ePWMxBStatus=off  ePWMxBactionLogic1=Set  ePWMxBactionLogic2=Clear  ePWMxBactionLogic3=Do nothing  ePWMxBactionLogic4=Do nothing  ePWMxBactionLogic5=Clear  ePWMxBactionLogic6=Set  ePWMxBLoadMode=Load on counter equals to zero (CTR=Zero)  ePWMxBCSFenable=off  ePWMxBCSFvalue=Forcing disable  ePWMxBSFreload=Zero  ePWNxBOutWay=off  ePWMxLINKCMPA=Not Linked  CMPAUnits=Clock cycles  CMPASource=Input port  CMPAValue_per=50  CMPAValue_clk=32000  enCMPAshadow=Counter equals to zero  ePWMxLINKCMPB=Not Linked  CMPBUnits=Clock cycles  CMPBSource=Specify via dialog  CMPBValue_per=50  CMPBValue_clk=32000  enCMPBshadow=Counter equals to zero  ePWMxLINKCMPC=Not Linked  CMPCUnits=Clock cycles  CMPCSource=Specify via dialog  CMPCValue_per=50  CMPCValue_clk=32000  enCMPCshadow=Counter equals to zero  ePWMxLINKCMPD=Not Linked  CMPDUnits=Clock cycles  CMPDSource=Specify via dialog  CMPDValue_per=50  CMPDValue_clk=32000  enCMPDshadow=Counter equals to zero  enableDBePWMxA=off  enableDBePWMxB=off  enhalfcycle=off  DBpolarity=Active high (AH)  DBedgeDelay=Positive  DBSource_ePWMxA=ePWMxA  DBSource_ePWMxB=ePWMxA  DBperiodSource=Specify via dialog  REDperiod=0  FEDperiod=0  adcstartModuleA=off  adcrequestEventA=First event  adcstartEventA=Digital Compare Module A Event 1 start of conversion (DCAEVT1.soc)  adcstartEventA_type2=Digital Compare Module A Event 1 start of conversion (DCAEVT1.soc)  adcstartModuleB=off  adcrequestEventB=First event  adcstartEventB=Counter equals to zero (CTR=Zero)  adcstartEventB_type2=Counter equals to zero (CTR=Zero)  intEn=off  intPrd=First event  intSel=Counter equals to zero (CTR=Zero)  intSel_type2=Counter equals to zero (CTR=Zero)  hrpe=off  enHRPWM=off  HRPWM_LoadMode=Counter equals to period (CTR=PRD)  HRPWM_CTLMode=Duty or Period control mode  HRPWM_EDGMode=Both edge  hrpeb=off  enHRPWMB=off  HRPWM_LoadModeB=Counter equals to zero (CTR=ZERO)  HRPWM_CTLModeB=Duty or Period control mode  HRPWM_EDGModeB=Both edge  enSFO=on  enautoconv=on  chopperEnable=off  chopperFrequency=1  chopperFirstwidth=1  chopperDuty=12.5%  tripZonesource=Specify via dialog  tzselOSHT1=off  tzselOSHT2=off  tzselOSHT3=off  tzselOSHDCAEV1=off  tzselOSHDCBEV1=off  tzselCBC1=off  tzselCBC2=off  tzselCBC3=off  tzselCBCDCAEV2=off  tzselCBCDCBEV2=off  tzselOSHT4=off  tzselOSHT5=off  tzselOSHT6=off  tzselCBC4=off  tzselCBC5=off  tzselCBC6=off  enTzOstIntr=off  enTzCbcIntr=off  enTzDCAEVT1Intr=off  enTzDCAEVT2Intr=off  enTzDCBEVT1Intr=off  enTzDCBEVT2Intr=off  ePWMxAforced=No action  ePWMxBforced=No action  DCAEVT1forced=No action  DCBEVT1forced=No action  DCAEVT2forced=No action  DCBEVT2forced=No action  dcah=Trip Zone 1 input (TZ1)  dcal=Trip Zone 2 input (TZ2)  dcbh=Trip Zone 1 input (TZ1)  dcbl=Trip Zone 2 input (TZ2)  dcah_type2=GPTRIP1SEL/(TZ1)  dcal_type2=GPTRIP2SEL/(TZ2)  dcbh_type2=GPTRIP1SEL/(TZ1)  dcbl_type2=GPTRIP2SEL/(TZ2)  gendcaevt1=Event disabled  gendcaevt2=Event disabled  gendcbevt1=Event disabled  gendcbevt2=Event disabled  dcaevt1src=DCAEVT1 with sync  dcaevt2src=DCAEVT2 with sync  dcbevt1src=DCBEVT1 with sync  dcbevt2src=DCBEVT2 with sync  pulsesel=Counter equals to zero (CTR=Zero)  blankinv=off  blankoffset=0  blankwidth=0  evsrcsel=Filtered version of DCAEVT1 (DCAEVT1FILT)  encape=off  PwmType=C2000_Type4
      settings: SourceProductName=Embedded Coder Support Package for Texas Instruments C2000 Processors
  wires:
  Gain/1 -> ePWM/1
  Constant4/1 -> DIR2/1
  Constant2/1 -> DIR1/1
  Bus Element In1/1 -> ENA2/1, ENA1/1
  Gain1/1 -> ePWM1/1
  Gain3/1 -> ePWM3/1
  Bus Element In3/1 -> ENA4/1, ENA3/1
  Constant8/1 -> DIR3/1
  Constant9/1 -> DIR4/1
  Gain2/1 -> ePWM2/1
  Saturation/1 -> Gain/1
  Saturation1/1 -> Gain1/1
  Saturation2/1 -> Gain2/1
  Saturation3/1 -> Gain3/1
  Bus Element In7/1 -> Saturation2/1
  Bus Element In6/1 -> Saturation3/1
  Bus Element In2/1 -> Saturation/1
  Bus Element In/1 -> Saturation1/1

== system rc_coder/Receive ==
  C28x Hardware Interrupt2 : c2000lib/Scheduling/C28x Hardware Interrupt  irqnumbers=[9]  pienumbers=[3]  irqpriorities=[30]  irqpreempts=[0]  showinput=off  dspchiptype=C280X
      settings: SourceProductName=Embedded Coder Support Package for Texas Instruments C2000 Processors  SourceProductBaseCode=TIC2000
  Rate Transition3 : RateTransition  Deterministic=off  OutPortSampleTimeOpt=Inherit
  Triggered Subsystem2 : Subsystem  TreatAsAtomicUnit=on
  RX : Outport
  wires:
  Rate Transition3/1 -> RX/1
  Triggered Subsystem2/1(Serial Command) -> Rate Transition3/1
  C28x Hardware Interrupt2/1 -> Triggered Subsystem2/Trigger

== system rc_coder/Sensing ==
  Current Measurement : Subsystem
      mask Display: disp('Current Measurement');
  Incremental Encoder : Subsystem
      mask Display: disp('Incremental Encoder');
  Temperature Measurement : Subsystem
      mask Display: disp('Temperature Measurement');
  Bus Element Out : Outport  PortName=daq  Element=ENC
  Bus Element Out1 : Outport  PortName=daq  Element=T
  Bus Element Out2 : Outport  PortName=daq  Element=I
  wires:
  Incremental Encoder/1(OutBus) -> Bus Element Out/1
  Temperature Measurement/1(OutBus) -> Bus Element Out1/1
  Current Measurement/1(OutBus) -> Bus Element Out2/1

== system rc_coder/SerialCommInterface1 ==
  TX : Inport
  C28x Hardware Interrupt1 : c2000lib/Scheduling/C28x Hardware Interrupt  irqnumbers=[9]  pienumbers=[1]  irqpriorities=[30]  irqpreempts=[0]  showinput=off  dspchiptype=C280X
      settings: SourceProductName=Embedded Coder Support Package for Texas Instruments C2000 Processors  SourceProductBaseCode=TIC2000
  Rate Transition1 : RateTransition  Deterministic=off  OutPortSampleTimeOpt=Inherit
  Rate Transition2 : RateTransition  Deterministic=off
  Triggered Subsystem1 : Subsystem  TreatAsAtomicUnit=on
  RX : Outport
  wires:
  C28x Hardware Interrupt1/1 -> Triggered Subsystem1/Trigger
  Rate Transition1/1 -> RX/1
  Triggered Subsystem1/1(Serial Command) -> Rate Transition1/1
  Rate Transition2/1 -> Triggered Subsystem1/1(TX)
  TX/1 -> Rate Transition2/1

== system rc_coder/Transmit ==
  RX : Inport
  status : Inport  Port=2
  TX : Inport  Port=3
  DataFlowSwitch : Subsystem
  If : If  IfExpression=u1 == 1  ShowElse=off
  If Action Subsystem : Subsystem  TreatAsAtomicUnit=on
  Rate Transition2 : RateTransition  Deterministic=off
  wires:
  If/1 -> If Action Subsystem/Action
  Rate Transition2/1 -> If Action Subsystem/3(data)
  TX/1 -> Rate Transition2/1
  status/1 -> DataFlowSwitch/1(status), If Action Subsystem/2(status)
  DataFlowSwitch/1(switch) -> If/1
  RX/1 -> If Action Subsystem/1(received)

== system rc_coder/Controller/Default ==
  Action Port : ActionPort  ActionPortLabel=default:
  Constant : Constant  Value=0  OutDataTypeStr=single
  Constant1 : Constant  Value=0  OutDataTypeStr=single
  Out1 : Outport
  Out2 : Outport  Port=2
  Out3 : Outport  Port=3
  Out4 : Outport  Port=4
  valve : Outport  Port=5
  wires:
  Constant/1 -> Out4/1, Out3/1, Out2/1, Out1/1
  Constant1/1 -> valve/1

== system rc_coder/Controller/PWM Mode ==
  Cmd : Inport
  Action Port : ActionPort  ActionPortLabel=case [ 56 ]:
  Bus Selector : BusSelector  OutputSignals=Cmd1,Cmd2,Cmd3,Cmd4
  Constant : Constant  Value=0  OutDataTypeStr=single
  s1 : Outport
  s2 : Outport  Port=2
  s3 : Outport  Port=3
  s4 : Outport  Port=4
  valve : Outport  Port=5
  wires:
  Cmd/1 -> Bus Selector/1
  Bus Selector/2 -> s2/1  "<Cmd2>"
  Bus Selector/4 -> s4/1  "<Cmd4>"
  Bus Selector/3 -> s3/1  "<Cmd3>"
  Bus Selector/1 -> s1/1  "<Cmd1>"
  Constant/1 -> valve/1

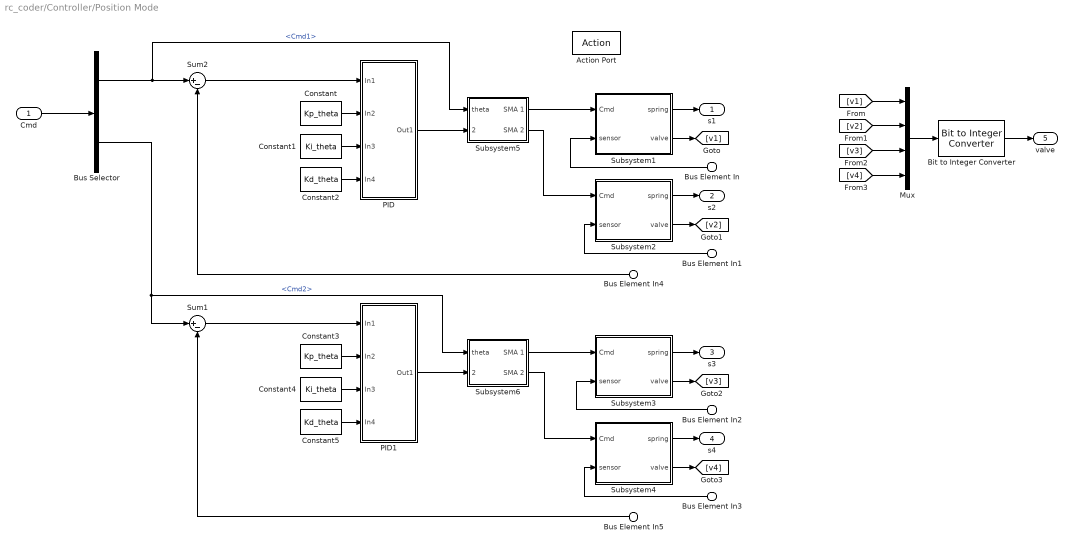
== system rc_coder/Controller/Position Mode ==
  Cmd : Inport
  Bus Element In : Inport  Port=2  PortName=feedback  Element=T.T1
  Bus Element In1 : Inport  Port=2  PortName=feedback  Element=T.T2
  Bus Element In2 : Inport  Port=2  PortName=feedback  Element=T.T3
  Bus Element In3 : Inport  Port=2  PortName=feedback  Element=T.T4
  Bus Element In4 : Inport  Port=2  PortName=feedback  Element=ENC.PosA
  Bus Element In5 : Inport  Port=2  PortName=feedback  Element=ENC.PosB
  Action Port : ActionPort  InitializeStates=reset  ActionPortLabel=case [ 53 ]:
  Bit to Integer Converter : commutil2/Bit to Integer Converter  nbits=4  bitOrder=MSB first  signedOutputValues=Unsigned  outDtype=Inherit via internal rule  outDtypeSigned=Inherit via internal rule
      settings: SourceProductName=Communications Toolbox
  Bus Selector : BusSelector  OutputSignals=Cmd1,Cmd2
  Constant : Constant  Value=Kp_theta
  Constant1 : Constant  Value=Ki_theta
  Constant2 : Constant  Value=Kd_theta
  Constant3 : Constant  Value=Kp_theta
  Constant4 : Constant  Value=Ki_theta
  Constant5 : Constant  Value=Kd_theta
  Mux : Mux
  PID : Subsystem
      mask Display:
      | disp('PID');
      | port_label('input', 1, 'e');
      | port_label('input', 2, 'Kp');
      | port_label('input', 3, 'Ki');
      | port_label('input', 4, 'Kd');
  PID1 : Subsystem
      mask Display:
      | disp('PID');
      | port_label('input', 1, 'e');
      | port_label('input', 2, 'Kp');
      | port_label('input', 3, 'Ki');
      | port_label('input', 4, 'Kd');
  Subsystem1 : Subsystem
  Subsystem2 : Subsystem
  Subsystem3 : Subsystem
  Subsystem4 : Subsystem
  Subsystem5 : Subsystem
  Subsystem6 : Subsystem
  Sum1 : Sum  Inputs=|+-
  Sum2 : Sum  Inputs=|+-
  s1 : Outport
  s2 : Outport  Port=2
  s3 : Outport  Port=3
  s4 : Outport  Port=4
  valve : Outport  Port=5
  wires:
  Subsystem4/2(valve) -> [v4]
  Subsystem3/2(valve) -> [v3]
  Bus Element In1/1 -> Subsystem2/2(sensor)
  Subsystem2/2(valve) -> [v2]
  Subsystem1/2(valve) -> [v1]
  Subsystem1/1(spring) -> s1/1
  Bus Element In/1 -> Subsystem1/2(sensor)
  Bit to Integer Converter/1 -> valve/1
  [v4] -> Mux/4
  [v3] -> Mux/3
  [v2] -> Mux/2
  [v1] -> Mux/1
  Mux/1 -> Bit to Integer Converter/1
  Bus Element In2/1 -> Subsystem3/2(sensor)
  Subsystem4/1(spring) -> s4/1
  Bus Element In3/1 -> Subsystem4/2(sensor)
  Subsystem3/1(spring) -> s3/1
  Subsystem2/1(spring) -> s2/1
  Cmd/1 -> Bus Selector/1
  Subsystem5/1(SMA 1) -> Subsystem1/1(Cmd)
  Subsystem5/2(SMA 2) -> Subsystem2/1(Cmd)
  PID/1(Out1) -> Subsystem5/2(delta_T)
  Sum2/1 -> PID/1(In1)
  Subsystem6/1(SMA 1) -> Subsystem3/1(Cmd)
  Subsystem6/2(SMA 2) -> Subsystem4/1(Cmd)
  PID1/1(Out1) -> Subsystem6/2(delta_T)
  Sum1/1 -> PID1/1(In1)
  Bus Selector/1 -> Sum2/1, Subsystem5/1(theta)  "<Cmd1>"
  Bus Selector/2 -> Subsystem6/1(theta), Sum1/1  "<Cmd2>"
  Bus Element In4/1 -> Sum2/2
  Bus Element In5/1 -> Sum1/2
  Constant/1 -> PID/2(In2)
  Constant1/1 -> PID/3(In3)
  Constant2/1 -> PID/4(In4)
  Constant3/1 -> PID1/2(In2)
  Constant4/1 -> PID1/3(In3)
  Constant5/1 -> PID1/4(In4)
